simulink model "template_Final_Project_MPC5643L"  (Simulink 7.8)
settings: Solver=FixedStepDiscrete  StartTime=0.0  StopTime=10.0  RelTol=1e-3
InitFcn:
  | parameters
values from neighbouring files (symbols this model uses):
  Ak = 100    [parameters.m]
  b = 100    [parameters.m]
  dT = 0.01    [parameters.m]
  H = 10    [ACCLogic_TestCase1.m]    (also in ACCLogic_TestCase2.m)
  Kd_PD = 0.03    [parameters.m]
  Kd_PID = 75    [parameters.m]
  Ki_PID = 0.002    [parameters.m]
  Kp_PD = 0.4    [parameters.m]
  Kp_PID = 550    [parameters.m]
  m = 2000    [parameters.m]
  V_Ki = 50    [parameters.m]
  V_Kp = 5000    [parameters.m]
undefined symbols (not defined in the file or in its folder): A10, A13, A14, AN1, AN12, B, B13, B4, B6, C6, D, D11, D4, DiscIntNeverNeededParam, F15, F3, F4, G4, H4, L3, M14, N15, P7, PA10, PA11, PA12, PA13, PA14, PA5, PA6, PA7, PA8, PA9, PB10, PB8, PC11, PC12, PC13, PC14, PC6, PD11, R10, R16, R8
libraries: Conv_Lib x50, rappid_564xl_ec_toolbox x36, Veh_Sim x9, simulink x3, U_of_M_5643_blockset x1
(part 1 of 2)
settings Model: Creator=lab  LastModifiedBy=cjzhang
settings DataIOCC: ExternalInput=off  InitialState=off  SaveOutput=off  SignalLogging=off  SaveTime=off
settings OptimizationCC: InlineParams=on  OptimizeModelRefInitCode=on  LifeSpan=1
settings DebuggingCC: InheritedTsInSrcMsg=none  SingleTaskRateTransMsg=error  UnconnectedInputMsg=error  UnconnectedOutputMsg=error  UnconnectedLineMsg=error  FrameProcessingCompatibilityMsg=error  UnknownTsInhSupMsg=error
settings HardwareCC: ProdLargestAtomicInteger=Long  ProdLargestAtomicFloat=Double  ProdIntDivRoundTo=Zero  ProdEndianess=BigEndian  ProdHWDeviceType=Motorola PowerPC
settings RTWCC: SystemTargetFile=rappid564xl.tlc  MakeCommand=rappid_564xl_make_rtw  TemplateMakefile=rappid_564xl_default_tmf  PostCodeGenCommand=rappid_analyzegencode(buildInfo)  Description=RAppID Toolbox MPC564xL Code Generation Target (rappid)  GenerateReport=on  ProcessScript=rappid564xl_make_rtw_hook  IncludeHyperlinkInReport=on  LaunchReport=on
settings CodeAppCC: IgnoreCustomStorageClasses=off
settings STFCustomTargetCC: TargetFunctionLibrary=C89/C90 (ANSI)  GeneratePreprocessorConditionals=Use local settings  CombineOutputUpdateFcns=on  SuppressErrorStatus=on  ERTCustomFileBanners=on  SupportContinuousTime=off  SupportNonInlinedSFcns=off  SystemTargetFile=rappid564xl.tlc
settings ERTTargetCC: TargetFunctionLibrary=C89/C90 (ANSI)  MultiwordLength=2048  ParMdlRefBuildCompliant=off  CompOptLevelCompliant=off  ConcurrentExecutionCompliant=off  SuppressErrorStatus=on  ERTFirstTimeCompliant=off  ModelStepFunctionPrototypeControlCompliant=off  CPPClassGenCompliant=off  ExtModeMexFile=noextcomm  InlinedParameterPlacement=NonHierarchical  ERTCustomFileTemplate=example_file_process.tlc  ConvertIfToSwitch=off  SuppressUnreachableDefaultCases=off

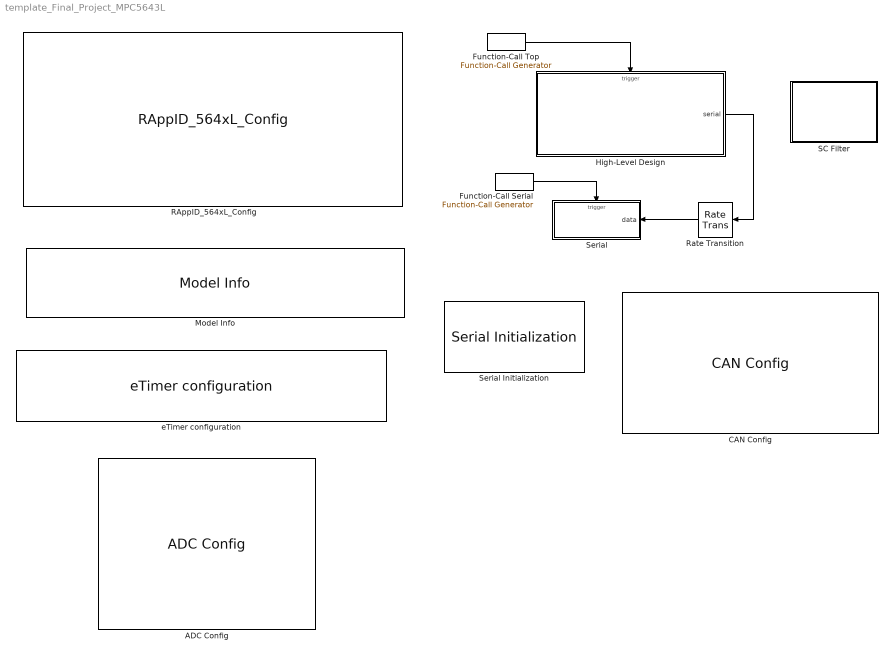
== system template_Final_Project_MPC5643L ==
  ADC Config : rappid_564xl_ec_toolbox/MPC564xL/Motor Control Blocks/ADC Config  adc_unit=0  adc_ctu=off  adc_owr=on  adc_wls=Left  adc_clk=on  adc_ack=on  adc_ctr0_inp=off  adc_ctr0_shft=10 - Avin = 0  adc_ctr0_cmp=01  adc_ctr0_samp=3  adc_ctr1_inp=off  adc_ctr1_cmp=01  adc_ctr1_samp=1  adc_ctr1_tsens=PTAT  adc_pscr_preval=V0  adc_pscr_preconv=off
  CAN Config : rappid_564xl_ec_toolbox/MPC564xL/Communication Blocks/CAN Config  Priority=1  can_unit=A  can_unit_v2=0  can_idam=A - One full ID (standard or extended) per filter element.  can_srx_dis=1 - Self reception disabled  can_presdiv=4  can_rjw=3  can_pseg1=5  can_pseg2=5  can_clk_src=0 - The CAN engine clock source is the oscillator clock  can_lpb=0 - Loop Back disabled  can_smp=0 - One sample is used to determine the bit value  can_boff_rec=0 - Automatic recovering from Bus Off state enabled  can_tsyn=0 - Timer Sync feature disabled  can_lbuf=0 - Buffer with highest priority is transmitted first  can_lom=0 - Listen Only Mode is deactivated  can_propseg=2
  Function-Call Serial : simulink/Ports & Subsystems/Function-Call Generator  sample_time=.05  numberOfIterations=1
  Function-Call Top : simulink/Ports & Subsystems/Function-Call Generator  sample_time=dT  numberOfIterations=1
  High-Level Design : Subsystem
  Model Info : simulink/Model-Wide Utilities/Model Info  InitialBlockCM=none  BlockCM=None  Frame=on  DisplayStringWithTags=|  HorizontalTextAlignment=Center  LeftAlignmentValue=0.5  SourceBlockDiagram=template_Final_Project_MPC5643L  TagMaxNumber=20
      | Model Notes:
      | 
      | You MUST change the CAN IDs whenever you change stations
      | 
      | First 2 buffers must be transmits
  RAppID_564xL_Config : rappid_564xl_ec_toolbox/MPC564xL/RAppID_564xL_Config  SystemClock=120  XTAL=40  MC_clock_60=12  MC_clock_80=16  MC_clock_120=10  SWG_clock_60=20  SWG_clock_80=13.334  SWG_clock_120=20  Compiler=CodeWarrior  MemTarget=FLASH  Part=MPC5643L  Package=144 LQFP  global_int_priority=10  base_tick_priority=11  sys_task_supress=off  exception_handlers=off  stored_mdl_name=adc_pit_block_new  freemaster_interface=Oops  freemaster_rx_pin="LINFlex_0 Rx Pin 116 : \"PB[3]\""  freemaster_tx_pin="LINFlex_0 Tx Pin 114 : \"PB[2]\""  freemaster_interface_1=Serial 0  freemaster_enable=on  freemaster_rate=115200  freemaster_tx0_pin=18 : B[2] : 114 : A14  freemaster_rx0_pin=19 : B[3] : 116 : B13  freemaster_tx1_pin=57 : D[9] : 26 : L3  freemaster_rx1_pin=29 : B[13] : 60 : R10  freemaster_can_channel=1CH  freemater_can_speed=500K  freemaster_can_msgig=0x7AA  ccp_interface=None  ccp_enable=off  ccp_can_channel=CH1 (MB 0 - 1)  ccp_can_speed=500K  ccp_can_cro_id=256  ccp_can_dto_id=257  ccp_dev_id=RappID  ccp_dev_addr=0  ccp_odt=3  ccp_daq=3  pil_enable=off  pil_bam=off  comport=4  pil_rate=115200  bam_password_def=on  bam_password=0xFEEDFACECAFEBEEF  bam_sa_cs=off  bam_start_address=0x0  bam_code_size=0x7000  cons_dspi=on  cons_can=on  cons_adc=on  cons_pwm=on  cons_ctu=on  cons_swg=on  cons_eTimer=on  cons_fm=on
  Rate Transition : RateTransition
  SC Filter : Subsystem
  Serial : Subsystem
  Serial Initialization : U_of_M_5643_blockset/Serial/Serial Initialization
  eTimer configuration : rappid_564xl_ec_toolbox/MPC564xL/Motor Control Blocks/eTimer configuration  SubModule=0  TimerChan=0  subMod=0  channel=0  CountMode=100 - Quadrature count mode using primary and secondary sources  CNTMODE=4  CountOnce=0 - Count repeatedly  ONCE=0  CountLength=0 - Continue counting to roll over  LENGTH=0  CountDirection=0 - Count up  DIR=0  OutputEnable=0 - The external pin is configured as an input  OEN=0  CoChanInit=00 - Other channels cannot force re-initialization of this channel  COINIT=0  StopAction=0 - Output enable is unaffected by stop mode  STPEN=0  ReloadOnCapt=00 - Do not reload the counter on a capture event  ROC=0  PrimarySource=00000 - Counter #0 input pin  PRISRC=0  PrimSrcPol=0 - True polarity  PIPS=0  SecondarySource=00001 - Counter #1 input pin  SECSRC=1  SecSrcPol=0 - True polarity  SIPS=0  FILT_CNT=0  FILT_PER=0  FILT=0  OutputMode=0000 - Software controlled  OUTMODE=0  OutputPol=0 - True polarity  OPS=0  MasterMode=0 - Disable broadcast of this channel output  MSTR=0  ForcedOutVal=0  VAL=0  CoForce=0 - Other channels cannot force this channel output  COFRC=0  CompLoad1=000 - COMP1 is never preload  CLC1=0  CompLoad2=000 - COMP2 is never preload  CLC2=0  CompareMode="00 - COMP1 and COMP2  are used when the counter is counting up"  CMPMODE=0  CaptMode1=00 - Capture disabled  CPT1MODE=0  CaptMode2=00 - Capture disabled  CPT2MODE=0  OneShCaptMode=0 - Free running mode is selected  ONESHOT=0  CaptFIFO=0  CFWM=0  CNTRinit=0  COMP1init=0  COMP2init=0  mod0ch0pin="0   : PA0  : [ 73 ] : [ T14 ]  input/output"  mod0ch1pin="1   : PA1  : [ 74 ] : [ R14 ]  input/output"  mod0ch2pin=None  mod0ch3pin=None  mod0ch4pin=None  mod0ch5pin=None  mod1ch0pin=None  mod1ch1pin=None  mod1ch2pin=None  mod1ch3pin=None  mod1ch4pin=None  mod1ch5pin=None  mod2ch0pin=None  mod2ch1pin=None  mod2ch2pin=None  mod2ch3pin=None  mod2ch4pin=None  mod2ch5pin=None  pcrNum0=0  pcrNum1=1  pcrNum2=255  pcrNum3=255  pcrNum4=255  pcrNum5=255  TCFIE=off  TCF1IE=off  TCF2IE=off  TOFIE=off  IELFIE=off  IEHFIE=off  ICF1IE=off  ICF2IE=off  INTDMA=0
  wires:
  Function-Call Serial/1 -> Serial/Trigger
  Rate Transition/1 -> Serial/1(data)
  Function-Call Top/1 -> High-Level Design/Trigger
  High-Level Design/1(serial) -> Rate Transition/1

== system template_Final_Project_MPC5643L/High-Level Design ==
  Trigger : TriggerPort  TriggerType=function-call
  Automatic Cruise Control : Subsystem
  Automatic Steering : Subsystem
  Inputs : Subsystem
  Outputs : Subsystem
  Unit Delay : UnitDelay  SampleTime=-1
  Vehicle Model : Subsystem
  serial : Outport
  wires:
  Outputs/1(x,y,psi (Cars 1 - 6)) -> serial/1
  Vehicle Model/3(u  (This Car)) -> Outputs/3(u (This Car))
  Inputs/1(s,n,psi,us (Cars 1 - 6)) -> Outputs/1(s,n,psi,us (Cars 1 - 6)), Automatic Cruise Control/1(s,n,psi,us (Cars 1 - 6))
  Vehicle Model/2(s,n,psi,us (This Car)) -> Outputs/2(s,n,psi,us (This Car)), Unit Delay/1
  Automatic Steering/1(Auto Torque) -> Outputs/5(Auto torque)
  Inputs/3(Cruise Control Speed) -> Automatic Cruise Control/3(Cruise Control Speed)
  Inputs/2(ACC_enable) -> Automatic Cruise Control/2("ACC_enable ")
  Inputs/4(Steering Angle (delta)) -> Automatic Cruise Control/4(Steering Angle (delta)), Automatic Steering/3(delta)
  Inputs/5(Throttle (Fd)) -> Automatic Cruise Control/5(Throttle (Fd))
  Inputs/6(Automatic Steering_enable) -> Automatic Steering/1(Automatic Steering_enable)
  Vehicle Model/1(Self-aligning torque) -> Outputs/4(Self-aligning torque)
  Unit Delay/1 -> Automatic Cruise Control/6(s,n,psi,us (This Car)), Automatic Steering/2(s,n,psi,us (This Car))
  Automatic Cruise Control/1(Force) -> Vehicle Model/1("Force ")
  Automatic Cruise Control/2(delta) -> Vehicle Model/2(delta)

== system template_Final_Project_MPC5643L/SC Filter ==
  Constant1 : Constant  Value=1e6  OutDataTypeStr=uint32
  Constant2 : Constant  Value=0  OutDataTypeStr=uint32
  Constant3 : Constant  Value=50  OutDataTypeStr=uint32
  Simple PWM Output : rappid_564xl_ec_toolbox/MPC564xL/Motor Control Blocks/Simple PWM Output  Priority=1  pwmModule=0  pwmMod=0  SubModule=1  subMod=1  InitFreq=1000000  resolution=1 %  resValue=1  InitDutyA=0  InitDutyB=50  align=A B - edge aligned  PhaseShift_A=0  PhaseShift=0  Phase_A=0  Phase_B=0  centered=0  DoubleS=off  doubleSw=off  debugSw=off  debug_mode=0  pin_A0=None  pin_B0=None  pin_X0=None  pin_A1=None  pin_B1="38  : PC6  : [ 142 ] : [ D4 ]"  pin_X1=None  pin_A2=None  pin_B2=None  pin_X2=None  pin_A3=None  pin_B3=None  pin_X3=None  pin1_A0=None  pin1_B0=None  pin1_X0=None  pin1_A1=None  pin1_B1=None  pin1_X1=None  pin1_A2=None  pin1_B2=None  pin1_X2=None  pin1_A3=None  pin1_B3=None  pin1_X3=None  pcrNumA=255  pcrNumB=38  pcrNumX=255  polA=off  polB=off  polX=off  octrl=0  syncFrom0=off  masterSync=0  outVal0=off  outVal1=off  outVal2=off  outVal3=off  outVal4=on  outVal5=on  outTrig=48
  wires:
  Constant1/1 -> Simple PWM Output/1
  Constant2/1 -> Simple PWM Output/2
  Constant3/1 -> Simple PWM Output/3

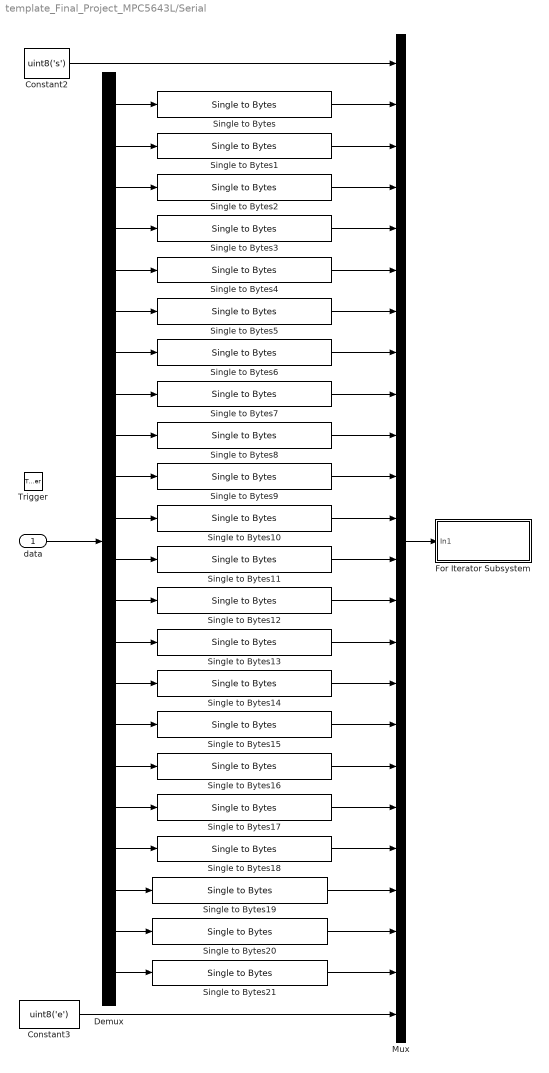
== system template_Final_Project_MPC5643L/Serial ==
  data : Inport
  Trigger : TriggerPort  TriggerType=function-call
  Constant2 : Constant  Value=uint8('s')  OutDataTypeStr=uint8
  Constant3 : Constant  Value=uint8('e')  OutDataTypeStr=uint8
  Demux : Demux  Outputs=22
  For Iterator Subsystem : Subsystem
  Mux : Mux  Inputs=24
  Single to Bytes{,1..21} (22 alike) : Conv_Lib/Single to Bytes
  wires:
  Constant2/1 -> Mux/1
  Single to Bytes/1 -> Mux/2
  Single to Bytes1/1 -> Mux/3
  Single to Bytes2/1 -> Mux/4
  Single to Bytes3/1 -> Mux/5
  Single to Bytes4/1 -> Mux/6
  Single to Bytes5/1 -> Mux/7
  Single to Bytes6/1 -> Mux/8
  Single to Bytes7/1 -> Mux/9
  Single to Bytes8/1 -> Mux/10
  Single to Bytes9/1 -> Mux/11
  Single to Bytes10/1 -> Mux/12
  Single to Bytes11/1 -> Mux/13
  Single to Bytes12/1 -> Mux/14
  Single to Bytes13/1 -> Mux/15
  Single to Bytes15/1 -> Mux/17
  Single to Bytes16/1 -> Mux/18
  Single to Bytes17/1 -> Mux/19
  Mux/1 -> For Iterator Subsystem/1(In1)
  Demux/1 -> Single to Bytes/1
  Demux/2 -> Single to Bytes1/1
  Demux/3 -> Single to Bytes2/1
  Demux/4 -> Single to Bytes3/1
  Demux/5 -> Single to Bytes4/1
  Demux/6 -> Single to Bytes5/1
  Demux/7 -> Single to Bytes6/1
  Demux/8 -> Single to Bytes7/1
  Demux/9 -> Single to Bytes8/1
  Demux/10 -> Single to Bytes9/1
  Demux/11 -> Single to Bytes10/1
  Demux/12 -> Single to Bytes11/1
  Demux/13 -> Single to Bytes12/1
  Demux/14 -> Single to Bytes13/1
  Demux/15 -> Single to Bytes14/1
  Demux/16 -> Single to Bytes15/1
  Demux/17 -> Single to Bytes16/1
  Demux/18 -> Single to Bytes17/1
  data/1 -> Demux/1
  Single to Bytes14/1 -> Mux/16
  Demux/19 -> Single to Bytes18/1
  Demux/20 -> Single to Bytes19/1
  Demux/21 -> Single to Bytes20/1
  Demux/22 -> Single to Bytes21/1
  Single to Bytes18/1 -> Mux/20
  Single to Bytes19/1 -> Mux/21
  Single to Bytes20/1 -> Mux/22
  Single to Bytes21/1 -> Mux/23
  Constant3/1 -> Mux/24

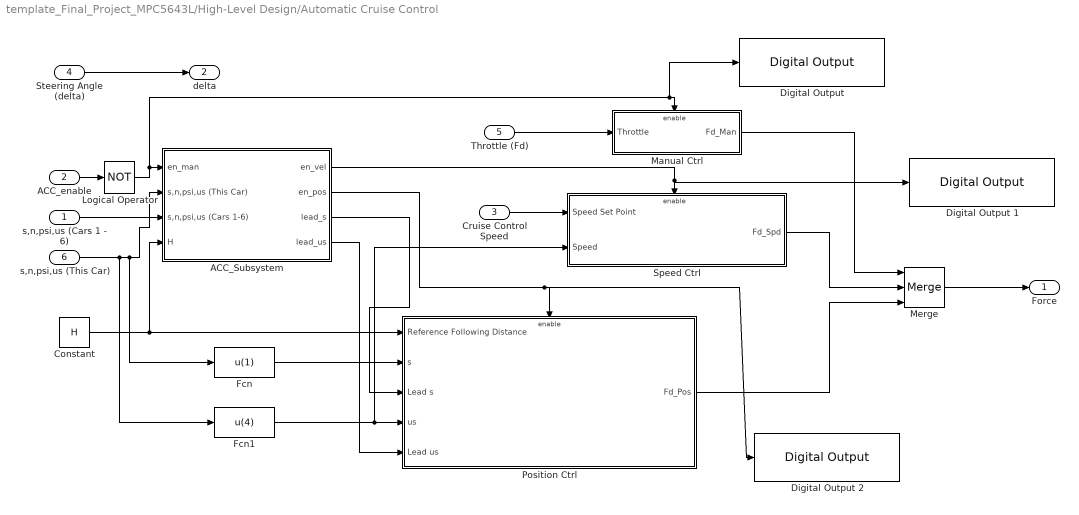
== system template_Final_Project_MPC5643L/High-Level Design/Automatic Cruise Control ==
  s,n,psi,us (Cars 1 - 6) : Inport
  "ACC_enable " : Inport  Port=2
  Cruise Control Speed : Inport  Port=3
  Steering Angle (delta) : Inport  Port=4
  Throttle (Fd) : Inport  Port=5
  s,n,psi,us (This Car) : Inport  Port=6
  ACC_Subsystem : Subsystem
  Constant : Constant  Value=H  OutDataTypeStr=single
  "Digital Output " : rappid_564xl_ec_toolbox/MPC564xL/General Purpose Blocks/Digital Output   gpio_outputs="43  : PC11 : [ 80 ] : [ M14 ]"  pinNum=[ 80 ]  pcrNum=43
  Digital Output 1 : rappid_564xl_ec_toolbox/MPC564xL/General Purpose Blocks/Digital Output   gpio_outputs="44  : PC12 : [ 82 ] : [ N15 ]"  pinNum=[ 82 ]  pcrNum=44
  Digital Output 2 : rappid_564xl_ec_toolbox/MPC564xL/General Purpose Blocks/Digital Output   gpio_outputs="45  : PC13 : [ 101 ] : [ F15 ]"  pinNum=[ 101 ]  pcrNum=45
  Fcn : Fcn  Expr=u(1)
  Fcn1 : Fcn  Expr=u(4)
  Logical Operator : Logic  Operator=NOT  AllPortsSameDT=off  OutDataTypeStr=boolean
  Manual Ctrl : Subsystem  TreatAsAtomicUnit=on
  Merge : Merge  Inputs=3
  Position Ctrl : Subsystem  TreatAsAtomicUnit=on
  Speed Ctrl : Subsystem  TreatAsAtomicUnit=on
  Force : Outport
  delta : Outport  Port=2
  wires:
  Steering Angle (delta)/1 -> delta/1
  Cruise Control Speed/1 -> Speed Ctrl/1(Speed Set Point)
  Speed Ctrl/1(Fd_Spd) -> Merge/2
  Position Ctrl/1(Fd_Pos) -> Merge/3
  Fcn/1 -> Position Ctrl/2(s)
  Fcn1/1 -> Position Ctrl/4(us), Speed Ctrl/2(Speed)
  Constant/1 -> Position Ctrl/1(Reference Following Distance), ACC_Subsystem/4(H)
  Throttle (Fd)/1 -> Manual Ctrl/1(Throttle)
  Manual Ctrl/1(Fd_Man) -> Merge/1
  Merge/1 -> Force/1
  "ACC_enable "/1 -> Logical Operator/1
  s,n,psi,us (This Car)/1 -> ACC_Subsystem/2(s,n,psi,us (This Car)), Fcn/1, Fcn1/1
  s,n,psi,us (Cars 1 - 6)/1 -> ACC_Subsystem/3(s,n,psi,us (Cars 1-6))
  Logical Operator/1 -> ACC_Subsystem/1(en_man), Manual Ctrl/Enable, "Digital Output "/1
  ACC_Subsystem/2(en_pos) -> Position Ctrl/Enable, Digital Output 2/1
  ACC_Subsystem/3(lead_s) -> Position Ctrl/3(Lead s)
  ACC_Subsystem/4(lead_us) -> Position Ctrl/5(Lead us)
  ACC_Subsystem/1(en_vel) -> Speed Ctrl/Enable, Digital Output 1/1

== system template_Final_Project_MPC5643L/High-Level Design/Automatic Steering ==
  Automatic Steering_enable : Inport
  s,n,psi,us (This Car) : Inport  Port=2
  delta : Inport  Port=3
  Automatic Steering : Subsystem  TreatAsAtomicUnit=on
  Constant1 : Constant  Value=0  OutDataTypeStr=single
  Digital Output 3 : rappid_564xl_ec_toolbox/MPC564xL/General Purpose Blocks/Digital Output   gpio_outputs="46  : PC14 : [ 103 ] : [ E15 ]"  pinNum=[ 103 ]  pcrNum=46
  Switch : Switch  Criteria=u2 > Threshold
  Auto Torque : Outport
  wires:
  Automatic Steering_enable/1 -> Automatic Steering/Enable, Switch/2, Digital Output 3/1
  s,n,psi,us (This Car)/1 -> Automatic Steering/1(s,n,psi,us (This Car))
  delta/1 -> Automatic Steering/2(delta)
  Constant1/1 -> Switch/3
  Automatic Steering/1(auto_torque) -> Switch/1
  Switch/1 -> Auto Torque/1

== system template_Final_Project_MPC5643L/High-Level Design/Inputs ==
  ADC Channel1 : rappid_564xl_ec_toolbox/MPC564xL/Motor Control Blocks/ADC Channel  adc_unit=0  adc_chan0=older  adc_chan0_v2=24 : PB8 : [47] : [P7] : AN1  adc_chan1=older  adc_chan1_v2=26 : PB10 : [53] : [R8] : AN12  simulate=off  interrupt=off  adc_mode=Normal  adc_presample=off
  Constant1 : Constant  Value=50  OutDataTypeStr=single
  Digital Input : rappid_564xl_ec_toolbox/MPC564xL/General Purpose Blocks/Digital Input  gpio_outputs="13  : PA13 : [ 136 ] : [ C6 ]"  pinNum=[ 136 ]  pcrNum=13
  Digital Input1 : rappid_564xl_ec_toolbox/MPC564xL/General Purpose Blocks/Digital Input  gpio_outputs="14  : PA14 : [ 143 ] : [ B4 ]"  pinNum=[ 143 ]  pcrNum=14
  Haptic Wheel Input : Subsystem
  Other Cars : Subsystem
  Read 8 bits : Subsystem
  Sum : Sum  Inputs=+|-
  s,n,psi,us (Cars 1 - 6) : Outport
  ACC_enable : Outport  Port=2
  Cruise Control Speed : Outport  Port=3
  Steering Angle (delta) : Outport  Port=4
  Throttle (Fd) : Outport  Port=5
  Automatic Steering_enable : Outport  Port=6
  wires:
  Digital Input1/1 -> Automatic Steering_enable/1
  Other Cars/1(s,n,psi,us (Car 1 - 6)) -> s,n,psi,us (Cars 1 - 6)/1
  Digital Input/1 -> ACC_enable/1
  Haptic Wheel Input/1(Haptic Wheel Position (radians)) -> Steering Angle (delta)/1
  Read 8 bits/1(8 bits) -> Cruise Control Speed/1
  ADC Channel1/1 -> Sum/1
  Sum/1 -> Throttle (Fd)/1
  Constant1/1 -> Sum/2

== system template_Final_Project_MPC5643L/High-Level Design/Outputs ==
  s,n,psi,us (Cars 1 - 6) : Inport
  s,n,psi,us (This Car) : Inport  Port=2
  u (This Car) : Inport  Port=3
  Self-aligning torque : Inport  Port=4
  Auto torque : Inport  Port=5
  Extract x,y,psi : Subsystem
  Extract x,y,psi (Cars 1 - 6) : Subsystem
  Mux : Mux  Inputs=3
  Subsystem : Subsystem
  Sum : Sum  Inputs=+|+
  Tx CAN : Subsystem
  x,y,psi (Cars 1 - 6) : Outport
  wires:
  s,n,psi,us (Cars 1 - 6)/1 -> Extract x,y,psi (Cars 1 - 6)/1(s,n,psi,us (Cars 1 - 6))
  s,n,psi,us (This Car)/1 -> Extract x,y,psi/1(s,n,psi,us), Tx CAN/1(s,n,psi,us)
  Extract x,y,psi/1(x,y,psi) -> Mux/1
  Mux/1 -> x,y,psi (Cars 1 - 6)/1
  u (This Car)/1 -> Mux/2
  Extract x,y,psi (Cars 1 - 6)/1(x,y,psi (Cars 1 - 6)) -> Mux/3
  Self-aligning torque/1 -> Sum/1
  Auto torque/1 -> Sum/2
  Sum/1 -> Subsystem/1(Torque)

== system template_Final_Project_MPC5643L/High-Level Design/Vehicle Model ==
  "Force " : Inport
  delta : Inport  Port=2
  Gain : Gain  Gain=Ak
  Look up Forward Vector : Veh_Sim/Look up Forward Vector  SystemSampleTime=-1
  Mux : Mux
  Product : Product  RndMeth=Zero
  S-Function Builder : S-Function  InitFcn=try, set_param(gcb,'FunctionName','us_calc'), end  FunctionName=us_calc  SFunctionModules=us_calc_wrapper  WizardData=DataTag0  EnableBusSupport=off  mask(S-Function Builder){}
      mask help: Simulink:masks:SFunctionBuilder_MD
      mask init:
      | val = [[.9  0.75 0.75 1 1 .9 .9 1]',[1 1 0.75 0.75 .9 .9 1 .9]'];try , sys = get_param(gcb,'SfunBuilderFcnName');if isempty(sys), sys = get_param(gcb,'FunctionName'); end,catch, sys = get_param(gcb,'FunctionName'); end
      settings: CopyFcn=set_param(gcbh,'LinkStatus','none')  PreSaveFcn=try, set_param(gcb,'FunctionName','us_calc'), end  OpenFcn=sfunctionwizard(gcbh)
      mask Display: plot(val(:,1),val(:,2)),disp(sys), port_label('input',1,'delta'), port_label('input',2,'psi'), port_label('input',3,'fx'), port_label('input',4,'fy'), port_label('input',5,'u'), port_label('output',1,'us')
  Vehicle Dynamics : Subsystem  TreatAsAtomicUnit=on
  x,y to s,n : Veh_Sim/x,y to s,n  SystemSampleTime=-1
  Self-aligning torque : Outport
  s,n,psi,us (This Car) : Outport  Port=2
  u  (This Car) : Outport  Port=3
  wires:
  "Force "/1 -> Vehicle Dynamics/1(Fd)
  delta/1 -> Vehicle Dynamics/2(delta), Product/2, S-Function Builder/1
  Vehicle Dynamics/3(u) -> Product/1, u  (This Car)/1, S-Function Builder/5
  Gain/1 -> Self-aligning torque/1
  Product/1 -> Gain/1
  Vehicle Dynamics/1(x) -> x,y to s,n/1
  Vehicle Dynamics/2(y) -> x,y to s,n/2
  x,y to s,n/1 -> Mux/1, Look up Forward Vector/1
  x,y to s,n/2 -> Mux/2
  Vehicle Dynamics/4(psi) -> Mux/3, S-Function Builder/2
  Look up Forward Vector/1 -> S-Function Builder/3
  Look up Forward Vector/2 -> S-Function Builder/4
  S-Function Builder/1 -> Mux/4
  Mux/1 -> s,n,psi,us (This Car)/1

== system template_Final_Project_MPC5643L/Serial/For Iterator Subsystem ==
  In1 : Inport
  Data Type Conversion : DataTypeConversion  OutDataTypeStr=uint8
  For Iterator : ForIterator  IterationLimit=91  IndexMode=Zero-based  IterationVariableDataType=int8
  Index Vector : MultiPortSwitch  DataPortOrder=Zero-based contiguous  Inputs=1  zeroidx=on
  S-Function : S-Function  FunctionName=SerialSend  EnableBusSupport=off
  wires:
  In1/1 -> Index Vector/2
  Index Vector/1 -> Data Type Conversion/1
  For Iterator/1 -> Index Vector/1
  Data Type Conversion/1 -> S-Function/1

== system template_Final_Project_MPC5643L/High-Level Design/Automatic Cruise Control/ACC_Subsystem ==
  en_man : Inport
  s,n,psi,us (This Car) : Inport  Port=2
  s,n,psi,us (Cars 1-6) : Inport  Port=3
  H : Inport  Port=4
  S-Function Builder : S-Function  InitFcn=try, set_param(gcb,'FunctionName','ACC_Logic'), end  FunctionName=ACC_Logic  SFunctionModules=ACC_Logic_wrapper  EnableBusSupport=off
      mask init: same as template_Final_Project_MPC5643L/High-Level Design/Vehicle Model/S-Function Builder
      settings: CopyFcn=set_param(gcbh,'LinkStatus','none')  PreSaveFcn=try, set_param(gcb,'FunctionName','ACC_Logic'), end  OpenFcn=sfunctionwizard(gcbh)
      mask Display: plot(val(:,1),val(:,2)),disp(sys), port_label('input',1,'en_man'), port_label('input',2,'s'), port_label('input',3,'u'), port_label('input',4,'H'), port_label('output',1,'en_vel'), port_label('output',2,'en_pos'), port_label('output',3,'lead_s'), port_label('output',4,'lead_us')
  Subsystem : Subsystem
  Subsystem1 : Subsystem
  en_vel : Outport
  en_pos : Outport  Port=2
  lead_s : Outport  Port=3
  lead_us : Outport  Port=4
  wires:
  en_man/1 -> S-Function Builder/1
  s,n,psi,us (This Car)/1 -> Subsystem/1(s,n,psi,us (This Car)), Subsystem1/1(s,n,psi,us (This Car))
  s,n,psi,us (Cars 1-6)/1 -> Subsystem/2(s,n,psi,us (Cars 1-6)), Subsystem1/2(s,n,psi,us (Cars 1-6))
  Subsystem/1(s) -> S-Function Builder/2
  S-Function Builder/2 -> en_pos/1
  S-Function Builder/3 -> lead_s/1
  Subsystem1/1(u) -> S-Function Builder/3
  H/1 -> S-Function Builder/4
  S-Function Builder/4 -> lead_us/1
  S-Function Builder/1 -> en_vel/1

== system template_Final_Project_MPC5643L/High-Level Design/Automatic Cruise Control/Manual Ctrl ==
  Throttle : Inport
  Enable : EnablePort
  Fd_Man : Outport
  wires:
  Throttle/1 -> Fd_Man/1  "desired speed"

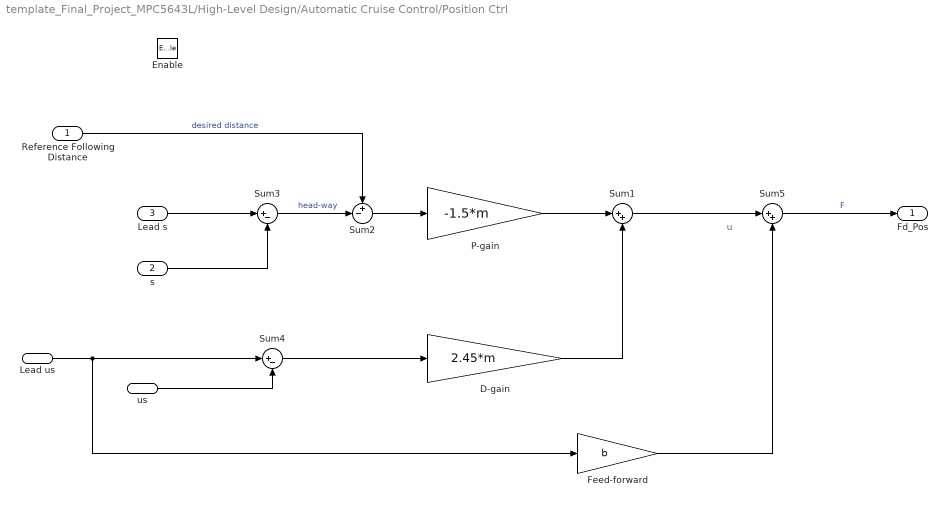
== system template_Final_Project_MPC5643L/High-Level Design/Automatic Cruise Control/Position Ctrl ==
  note: u
  Reference Following Distance : Inport
  s : Inport  Port=2
  Lead s : Inport  Port=3
  us : Inport  Port=4
  Lead us : Inport  Port=5
  Enable : EnablePort
  D-gain : Gain  Gain=2.45*m  SaturateOnIntegerOverflow=on  OutDataTypeStr=Inherit: Same as input  ParamDataTypeStr=Inherit: Same as input
  Feed-forward : Gain  Gain=b  SaturateOnIntegerOverflow=on  OutDataTypeStr=Inherit: Same as input  ParamDataTypeStr=Inherit: Same as input
  P-gain : Gain  Gain=-1.5*m  SaturateOnIntegerOverflow=on  OutDataTypeStr=Inherit: Same as input  ParamDataTypeStr=Inherit: Same as input
  Sum1 : Sum  Inputs=|++  SaturateOnIntegerOverflow=on
  Sum2 : Sum  Inputs=+-|  SaturateOnIntegerOverflow=on
  Sum3 : Sum  Inputs=|+-  SaturateOnIntegerOverflow=on
  Sum4 : Sum  Inputs=|+-  SaturateOnIntegerOverflow=on
  Sum5 : Sum  Inputs=|++  SaturateOnIntegerOverflow=on
  Fd_Pos : Outport
  wires:
  Sum1/1 -> Sum5/1
  Sum5/1 -> Fd_Pos/1  "F"
  Feed-forward/1 -> Sum5/2
  Sum4/1 -> D-gain/1
  Lead us/1 -> Feed-forward/1, Sum4/1
  us/1 -> Sum4/2
  D-gain/1 -> Sum1/2
  P-gain/1 -> Sum1/1
  Sum2/1 -> P-gain/1
  Sum3/1 -> Sum2/2  "head-way"
  Reference Following Distance/1 -> Sum2/1  "desired distance"
  s/1 -> Sum3/2
  Lead s/1 -> Sum3/1

== system template_Final_Project_MPC5643L/High-Level Design/Automatic Cruise Control/Speed Ctrl ==
  Speed Set Point : Inport
  Speed : Inport  Port=2
  Enable : EnablePort
  Gain : Gain  Gain=b  SaturateOnIntegerOverflow=on  OutDataTypeStr=Inherit: Same as input  ParamDataTypeStr=Inherit: Same as input
  PI : Subsystem
  Sum : Sum  Inputs=++|  SaturateOnIntegerOverflow=on
  Sum1 : Sum  Inputs=|+-  SaturateOnIntegerOverflow=on
  Fd_Spd : Outport
  wires:
  PI/1(U) -> Sum/2
  Gain/1 -> Sum/1
  Sum1/1 -> PI/1(Error)
  Speed/1 -> Sum1/2
  Speed Set Point/1 -> Sum1/1, Gain/1  "desired speed"
  Sum/1 -> Fd_Spd/1  "Fd"

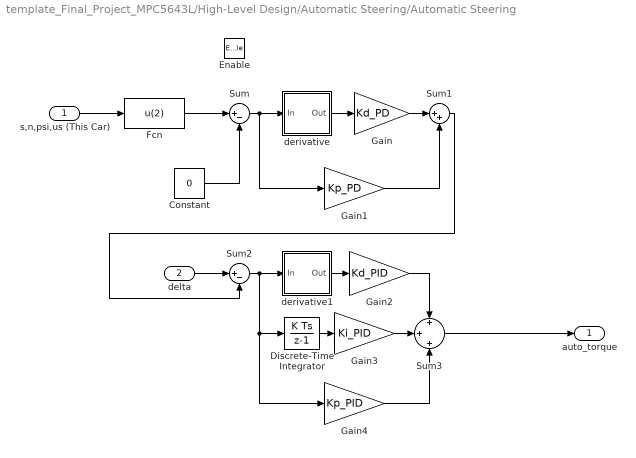
== system template_Final_Project_MPC5643L/High-Level Design/Automatic Steering/Automatic Steering ==
  s,n,psi,us (This Car) : Inport
  delta : Inport  Port=2
  Enable : EnablePort
  Constant : Constant  Value=0  OutDataTypeStr=single
  Discrete-Time Integrator : DiscreteIntegrator  SampleTime=-1  ICPrevOutput=DiscIntNeverNeededParam  ICPrevScaledInput=DiscIntNeverNeededParam
  Fcn : Fcn  Expr=u(2)
  Gain : Gain  Gain=Kd_PD
  Gain1 : Gain  Gain=Kp_PD
  Gain2 : Gain  Gain=Kd_PID
  Gain3 : Gain  Gain=Ki_PID
  Gain4 : Gain  Gain=Kp_PID
  Sum : Sum  Inputs=|+-
  Sum1 : Sum  Inputs=|++
  Sum2 : Sum  Inputs=|+-
  Sum3 : Sum  Inputs=+|+|+
  derivative : Subsystem
  derivative1 : Subsystem
  auto_torque : Outport
  wires:
  Sum/1 -> Gain1/1, derivative/1(In)
  Gain/1 -> Sum1/1
  Gain1/1 -> Sum1/2
  Sum2/1 -> Gain4/1, Discrete-Time Integrator/1, derivative1/1(In)
  Gain3/1 -> Sum3/2
  Gain2/1 -> Sum3/1
  Gain4/1 -> Sum3/3
  derivative1/1(Out) -> Gain2/1
  Discrete-Time Integrator/1 -> Gain3/1
  Constant/1 -> Sum/2
  derivative/1(Out) -> Gain/1
  Fcn/1 -> Sum/1
  s,n,psi,us (This Car)/1 -> Fcn/1
  Sum1/1 -> Sum2/2
  delta/1 -> Sum2/1
  Sum3/1 -> auto_torque/1

== system template_Final_Project_MPC5643L/High-Level Design/Inputs/Haptic Wheel Input ==
  Gain : Gain  Gain=-1
  Subsystem : Subsystem
  eTimer CNTR Register Read : rappid_564xl_ec_toolbox/MPC564xL/Motor Control Blocks/eTimer CNTR Register Read  SubModule=0  TimerChan=0  subMod=0  channel=0
  Haptic Wheel Position (radians) : Outport
  wires:
  eTimer CNTR Register Read/1 -> Subsystem/1(encoder counts)
  Subsystem/1(Haptic  Wheel  Position  (radians)) -> Gain/1
  Gain/1 -> Haptic Wheel Position (radians)/1

== system template_Final_Project_MPC5643L/High-Level Design/Inputs/Other Cars ==
  "0 for GSI vehicle only, 1 for ALL student vehicles" : Constant  OutDataTypeStr=single
  GSI Car : Subsystem
  GSI Car1 : Subsystem
  GSI Car2 : Subsystem
  GSI Car3 : Subsystem
  GSI Car4 : Subsystem
  GSI Car5 : Subsystem
  Mux1 : Mux  Inputs=6
  Switch : Switch  Criteria=u2 ~= 0
  s,n,psi,us (Car 1 - 6) : Outport
  wires:
  GSI Car/1(s,n,psi,us) -> Mux1/1
  Mux1/1 -> Switch/1, Switch/3
  Switch/1 -> s,n,psi,us (Car 1 - 6)/1
  "0 for GSI vehicle only, 1 for ALL student vehicles"/1 -> Switch/2
  GSI Car1/1(s,n,psi,us) -> Mux1/2
  GSI Car2/1(s,n,psi,us) -> Mux1/3
  GSI Car3/1(s,n,psi,us) -> Mux1/4
  GSI Car4/1(s,n,psi,us) -> Mux1/5
  GSI Car5/1(s,n,psi,us) -> Mux1/6

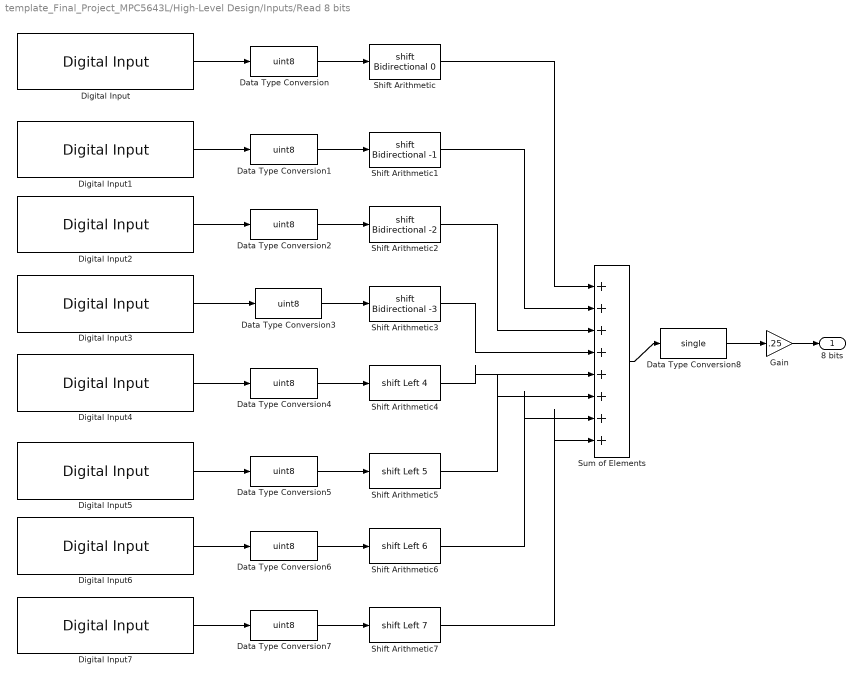
== system template_Final_Project_MPC5643L/High-Level Design/Inputs/Read 8 bits ==
  Data Type Conversion{,1..7} (8 alike) : DataTypeConversion  OutDataTypeStr=uint8
  Data Type Conversion8 : DataTypeConversion  OutDataTypeStr=single
  Digital Input : rappid_564xl_ec_toolbox/MPC564xL/General Purpose Blocks/Digital Input  gpio_outputs="5   : PA5  : [ 14 ] : [ H4 ]"  pinNum=[ 14 ]  pcrNum=5
  Digital Input1 : rappid_564xl_ec_toolbox/MPC564xL/General Purpose Blocks/Digital Input  gpio_outputs="6   : PA6  : [ 2 ] : [ G4 ]"  pinNum=[ 2 ]  pcrNum=6
  Digital Input2 : rappid_564xl_ec_toolbox/MPC564xL/General Purpose Blocks/Digital Input  gpio_outputs="7   : PA7  : [ 10 ] : [ F3 ]"  pinNum=[ 10 ]  pcrNum=7
  Digital Input3 : rappid_564xl_ec_toolbox/MPC564xL/General Purpose Blocks/Digital Input  gpio_outputs="8   : PA8  : [ 12 ] : [ F4 ]"  pinNum=[ 12 ]  pcrNum=8
  Digital Input4 : rappid_564xl_ec_toolbox/MPC564xL/General Purpose Blocks/Digital Input  gpio_outputs="9   : PA9  : [ 134 ] : [ B6 ]"  pinNum=[ 134 ]  pcrNum=9
  Digital Input5 : rappid_564xl_ec_toolbox/MPC564xL/General Purpose Blocks/Digital Input  gpio_outputs="10  : PA10  : [ 118 ] : [ A13 ]"  pinNum=[ 118 ]  pcrNum=10
  Digital Input6 : rappid_564xl_ec_toolbox/MPC564xL/General Purpose Blocks/Digital Input  gpio_outputs="11  : PA11 : [ 120 ] : [ D11 ]"  pinNum=[ 120 ]  pcrNum=11
  Digital Input7 : rappid_564xl_ec_toolbox/MPC564xL/General Purpose Blocks/Digital Input  gpio_outputs="12  : PA12 : [ 122 ] : [ A10 ]"  pinNum=[ 122 ]  pcrNum=12
  Gain : Gain  Gain=.25
  Shift Arithmetic : ArithShift
  Shift Arithmetic1 : ArithShift  BitShiftNumber=-1
  Shift Arithmetic2 : ArithShift  BitShiftNumber=-2
  Shift Arithmetic3 : ArithShift  BitShiftNumber=-3
  Shift Arithmetic4 : ArithShift  BitShiftNumber=4  BitShiftDirection=Left
  Shift Arithmetic5 : ArithShift  BitShiftNumber=5  BitShiftDirection=Left
  Shift Arithmetic6 : ArithShift  BitShiftNumber=6  BitShiftDirection=Left
  Shift Arithmetic7 : ArithShift  BitShiftNumber=7  BitShiftDirection=Left
  Sum of Elements : Sum  Inputs=|+|+|+|+|+|+|+|+  OutDataTypeStr=single
  8 bits : Outport
  wires:
  Digital Input/1 -> Data Type Conversion/1
  Digital Input1/1 -> Data Type Conversion1/1
  Digital Input2/1 -> Data Type Conversion2/1
  Digital Input3/1 -> Data Type Conversion3/1
  Data Type Conversion/1 -> Shift Arithmetic/1
  Data Type Conversion1/1 -> Shift Arithmetic1/1
  Data Type Conversion2/1 -> Shift Arithmetic2/1
  Data Type Conversion3/1 -> Shift Arithmetic3/1
  Shift Arithmetic1/1 -> Sum of Elements/2
  Shift Arithmetic2/1 -> Sum of Elements/3
  Shift Arithmetic3/1 -> Sum of Elements/4
  Digital Input4/1 -> Data Type Conversion4/1
  Digital Input5/1 -> Data Type Conversion5/1
  Digital Input6/1 -> Data Type Conversion6/1
  Digital Input7/1 -> Data Type Conversion7/1
  Data Type Conversion4/1 -> Shift Arithmetic4/1
  Data Type Conversion5/1 -> Shift Arithmetic5/1
  Data Type Conversion6/1 -> Shift Arithmetic6/1
  Data Type Conversion7/1 -> Shift Arithmetic7/1
  Shift Arithmetic4/1 -> Sum of Elements/5
  Shift Arithmetic5/1 -> Sum of Elements/6
  Shift Arithmetic6/1 -> Sum of Elements/7
  Shift Arithmetic7/1 -> Sum of Elements/8
  Shift Arithmetic/1 -> Sum of Elements/1
  Gain/1 -> 8 bits/1
  Sum of Elements/1 -> Data Type Conversion8/1
  Data Type Conversion8/1 -> Gain/1

== system template_Final_Project_MPC5643L/High-Level Design/Outputs/Extract x,y,psi ==
  s,n,psi,us : Inport
  Demux : Demux
  Mux : Mux  Inputs=3
  Terminator : Terminator
  s,n to x,y : Veh_Sim/s,n to x,y  SystemSampleTime=-1
  x,y,psi : Outport
  wires:
  Demux/1 -> s,n to x,y/1
  Demux/2 -> s,n to x,y/2
  s,n,psi,us/1 -> Demux/1
  s,n to x,y/1 -> Mux/1
  s,n to x,y/2 -> Mux/2
  Demux/3 -> Mux/3
  Demux/4 -> Terminator/1
  Mux/1 -> x,y,psi/1

== system template_Final_Project_MPC5643L/High-Level Design/Outputs/Extract x,y,psi (Cars 1 - 6) ==
  s,n,psi,us (Cars 1 - 6) : Inport
  Demux : Demux  Outputs=6
  Extract x,y,psi : Subsystem
  Extract x,y,psi1 : Subsystem
  Extract x,y,psi2 : Subsystem
  Extract x,y,psi3 : Subsystem
  Extract x,y,psi4 : Subsystem
  Extract x,y,psi5 : Subsystem
  Mux : Mux  Inputs=6
  x,y,psi (Cars 1 - 6) : Outport
  wires:
  Demux/1 -> Extract x,y,psi/1(s,n,psi,us)
  Extract x,y,psi/1(x,y,psi) -> Mux/1
  Demux/2 -> Extract x,y,psi1/1(s,n,psi,us)
  Extract x,y,psi1/1(x,y,psi) -> Mux/2
  Demux/3 -> Extract x,y,psi2/1(s,n,psi,us)
  Extract x,y,psi2/1(x,y,psi) -> Mux/3
  Demux/4 -> Extract x,y,psi3/1(s,n,psi,us)
  Extract x,y,psi3/1(x,y,psi) -> Mux/4
  Demux/5 -> Extract x,y,psi4/1(s,n,psi,us)
  Extract x,y,psi4/1(x,y,psi) -> Mux/5
  s,n,psi,us (Cars 1 - 6)/1 -> Demux/1
  Mux/1 -> x,y,psi (Cars 1 - 6)/1
  Extract x,y,psi5/1(x,y,psi) -> Mux/6
  Demux/6 -> Extract x,y,psi5/1(s,n,psi,us)

== system template_Final_Project_MPC5643L/High-Level Design/Outputs/Subsystem ==
  Torque : Inport
  Add : Sum
  Constant : Constant  Value=0.5  OutDataTypeStr=single
  Constant1 : Constant  Value=0.0003162  OutDataTypeStr=single
  Constant2 : Constant  Value=20000  OutDataTypeStr=uint32
  Constant3 : Constant  Value=100  OutDataTypeStr=single
  Constant4 : Constant  Value=0  OutDataTypeStr=uint32
  Product : Product  RndMeth=Zero
  Product1 : Product  OutDataTypeStr=uint32  RndMeth=Zero
  Saturation : Saturate  UpperLimit=0.76  LowerLimit=0.24
  Simple PWM Output : rappid_564xl_ec_toolbox/MPC564xL/Motor Control Blocks/Simple PWM Output  Priority=1  pwmModule=0  pwmMod=0  SubModule=0  subMod=0  InitFreq=20000  resolution=1 %  resValue=1  InitDutyA=0  InitDutyB=0  align=A - edge aligned B - phase shifted  PhaseShift_A=0  PhaseShift=0  Phase_A=0  Phase_B=0  centered=-1  DoubleS=off  doubleSw=off  debugSw=off  debug_mode=0  pin_A0=None  pin_B0="59  : PD11 : [ 78 ] : [ R16 ]"  pin_X0=None  pin_A1=None  pin_B1=None  pin_X1=None  pin_A2=None  pin_B2=None  pin_X2=None  pin_A3=None  pin_B3=None  pin_X3=None  pin1_A0=None  pin1_B0=None  pin1_X0=None  pin1_A1=None  pin1_B1=None  pin1_X1=None  pin1_A2=None  pin1_B2=None  pin1_X2=None  pin1_A3=None  pin1_B3=None  pin1_X3=None  pcrNumA=255  pcrNumB=59  pcrNumX=255  polA=off  polB=off  polX=off  octrl=0  syncFrom0=off  masterSync=0  outVal0=off  outVal1=off  outVal2=on  outVal3=on  outVal4=on  outVal5=on  outTrig=60
  wires:
  Constant1/1 -> Product/2
  Torque/1 -> Product/1
  Product/1 -> Add/1
  Constant/1 -> Add/2
  Add/1 -> Saturation/1
  Constant2/1 -> Simple PWM Output/1
  Constant4/1 -> Simple PWM Output/4
  Saturation/1 -> Product1/1
  Product1/1 -> Simple PWM Output/2, Simple PWM Output/3
  Constant3/1 -> Product1/2

== system template_Final_Project_MPC5643L/High-Level Design/Outputs/Tx CAN ==
  s,n,psi,us : Inport
  CAN Transmit : rappid_564xl_ec_toolbox/MPC564xL/Communication Blocks/CAN Transmit  can_unit=A  can_unit_v2=0  can_buffer=0  can_id=45
  CAN Transmit1 : rappid_564xl_ec_toolbox/MPC564xL/Communication Blocks/CAN Transmit  can_unit=A  can_unit_v2=0  can_buffer=1  can_id=46
  Constant : Constant  Value=8  OutDataTypeStr=uint8
  Constant1 : Constant  Value=8  OutDataTypeStr=uint8
  Demux : Demux
  Mux : Mux  Inputs=2
  Mux1 : Mux  Inputs=2
  Single to Bytes{,1..3} (4 alike) : Conv_Lib/Single to Bytes
  wires:
  Constant1/1 -> CAN Transmit1/2
  Single to Bytes/1 -> Mux/1
  Single to Bytes1/1 -> Mux/2
  Single to Bytes2/1 -> Mux1/1
  Single to Bytes3/1 -> Mux1/2
  Mux/1 -> CAN Transmit/1
  Demux/1 -> Single to Bytes/1
  Demux/2 -> Single to Bytes1/1
  Demux/3 -> Single to Bytes3/1
  Demux/4 -> Single to Bytes2/1
  s,n,psi,us/1 -> Demux/1
  Constant/1 -> CAN Transmit/2
  Mux1/1 -> CAN Transmit1/1

== system template_Final_Project_MPC5643L/High-Level Design/Vehicle Model/Vehicle Dynamics ==
  Fd : Inport
  delta : Inport  Port=2
  Discrete-Time Integrator1 : DiscreteIntegrator  gainval=1  SampleTime=-1  ICPrevOutput=DiscIntNeverNeededParam  ICPrevScaledInput=DiscIntNeverNeededParam
  Discrete-Time Integrator2 : DiscreteIntegrator  gainval=1  SampleTime=-1  ICPrevOutput=DiscIntNeverNeededParam  ICPrevScaledInput=DiscIntNeverNeededParam
  Discrete-Time Integrator3 : DiscreteIntegrator  gainval=1  SampleTime=-1  ICPrevOutput=DiscIntNeverNeededParam  ICPrevScaledInput=DiscIntNeverNeededParam
  Discrete-Time Integrator4 : DiscreteIntegrator  gainval=1  SampleTime=-1  OutDataTypeStr=single  ICPrevOutput=DiscIntNeverNeededParam  ICPrevScaledInput=DiscIntNeverNeededParam
  Gain1 : Gain  Gain=1/m
  Gain4 : Gain  Gain=b
  S-Function Builder : S-Function  InitFcn=try, set_param(gcb,'FunctionName','vehicle_model'), end  FunctionName=vehicle_model  SFunctionModules=vehicle_model_wrapper  WizardData=DataTag1  EnableBusSupport=off  mask(S-Function Builder){}
      mask help: Simulink:masks:SFunctionBuilder_MD
      mask init: same as template_Final_Project_MPC5643L/High-Level Design/Vehicle Model/S-Function Builder
      settings: CopyFcn=set_param(gcbh,'LinkStatus','none')  PreSaveFcn=try, set_param(gcb,'FunctionName','vehicle_model'), end  OpenFcn=sfunctionwizard(gcbh)
      mask Display: plot(val(:,1),val(:,2)),disp(sys), port_label('input',1,'u'), port_label('input',2,'psi'), port_label('input',3,'delta'), port_label('output',1,'dotx'), port_label('output',2,'doty'), port_label('output',3,'dotpsi')
  Sum : Sum  Inputs=|+-
  x : Outport
  y : Outport  Port=2
  u : Outport  Port=3
  psi : Outport  Port=4
  wires:
  S-Function Builder/1 -> Discrete-Time Integrator1/1
  S-Function Builder/2 -> Discrete-Time Integrator2/1
  Sum/1 -> Gain1/1
  Gain1/1 -> Discrete-Time Integrator3/1
  Gain4/1 -> Sum/2
  Fd/1 -> Sum/1
  Discrete-Time Integrator3/1 -> u/1, S-Function Builder/1, Gain4/1
  Discrete-Time Integrator1/1 -> x/1
  Discrete-Time Integrator2/1 -> y/1
  S-Function Builder/3 -> Discrete-Time Integrator4/1
  Discrete-Time Integrator4/1 -> S-Function Builder/2, psi/1
  delta/1 -> S-Function Builder/3

== system template_Final_Project_MPC5643L/High-Level Design/Automatic Cruise Control/ACC_Subsystem/Subsystem ==
  s,n,psi,us (This Car) : Inport
  s,n,psi,us (Cars 1-6) : Inport  Port=2
  Fcn : Fcn  Expr=u(1)
  Fcn1 : Fcn  Expr=u(1)
  Fcn2 : Fcn  Expr=u(5)
  Fcn3 : Fcn  Expr=u(9)
  Fcn4 : Fcn  Expr=u(13)
  Fcn5 : Fcn  Expr=u(17)
  Fcn6 : Fcn  Expr=u(21)
  Mux1 : Mux  Inputs=7
  s : Outport
  wires:
  Fcn/1 -> Mux1/1
  Fcn4/1 -> Mux1/5
  Fcn3/1 -> Mux1/4
  Mux1/1 -> s/1
  Fcn5/1 -> Mux1/6
  Fcn2/1 -> Mux1/3
  Fcn1/1 -> Mux1/2
  s,n,psi,us (Cars 1-6)/1 -> Fcn3/1, Fcn4/1, Fcn5/1, Fcn6/1, Fcn2/1, Fcn1/1
  s,n,psi,us (This Car)/1 -> Fcn/1
  Fcn6/1 -> Mux1/7

== system template_Final_Project_MPC5643L/High-Level Design/Automatic Cruise Control/ACC_Subsystem/Subsystem1 ==
  s,n,psi,us (This Car) : Inport
  s,n,psi,us (Cars 1-6) : Inport  Port=2
  Fcn : Fcn  Expr=u(4)
  Fcn1 : Fcn  Expr=u(4)
  Fcn2 : Fcn  Expr=u(8)
  Fcn3 : Fcn  Expr=u(12)
  Fcn4 : Fcn  Expr=u(16)
  Fcn5 : Fcn  Expr=u(20)
  Fcn6 : Fcn  Expr=u(20)
  Mux1 : Mux  Inputs=7
  u : Outport
  wires:
  Fcn/1 -> Mux1/1
  Fcn4/1 -> Mux1/5
  Fcn3/1 -> Mux1/4
  Mux1/1 -> u/1
  Fcn5/1 -> Mux1/6
  Fcn2/1 -> Mux1/3
  Fcn1/1 -> Mux1/2
  s,n,psi,us (Cars 1-6)/1 -> Fcn3/1, Fcn4/1, Fcn5/1, Fcn6/1, Fcn2/1, Fcn1/1
  s,n,psi,us (This Car)/1 -> Fcn/1
  Fcn6/1 -> Mux1/7

== system template_Final_Project_MPC5643L/High-Level Design/Automatic Cruise Control/Speed Ctrl/PI ==
  Error : Inport
  Gain : Gain  Gain=V_Ki  SaturateOnIntegerOverflow=on  OutDataTypeStr=Inherit: Same as input  ParamDataTypeStr=Inherit: Same as input
  Gain1 : Gain  Gain=V_Kp  SaturateOnIntegerOverflow=on  OutDataTypeStr=Inherit: Same as input  ParamDataTypeStr=Inherit: Same as input
  My Discrete Integrator : Subsystem
  Sum : Sum  Inputs=|++  SaturateOnIntegerOverflow=on
  U : Outport
  wires:
  Sum/1 -> U/1
  Error/1 -> Gain1/1, Gain/1
  Gain1/1 -> Sum/2
  My Discrete Integrator/1(X) -> Sum/1
  Gain/1 -> My Discrete Integrator/1(X_dot)

== system template_Final_Project_MPC5643L/High-Level Design/Automatic Steering/Automatic Steering/derivative ==
  In : Inport
  Gain5 : Gain  Gain=1/dT
  Sum4 : Sum  Inputs=|+-
  Unit Delay : UnitDelay  SampleTime=-1
  Out : Outport
  wires:
  Sum4/1 -> Gain5/1
  Unit Delay/1 -> Sum4/2
  In/1 -> Sum4/1, Unit Delay/1
  Gain5/1 -> Out/1

== system template_Final_Project_MPC5643L/High-Level Design/Automatic Steering/Automatic Steering/derivative1 ==
  In : Inport
  Gain5 : Gain  Gain=1/dT
  Sum4 : Sum  Inputs=|+-
  Unit Delay : UnitDelay  SampleTime=-1
  Out : Outport
  wires:
  Sum4/1 -> Gain5/1
  Unit Delay/1 -> Sum4/2
  In/1 -> Sum4/1, Unit Delay/1
  Gain5/1 -> Out/1

== system template_Final_Project_MPC5643L/High-Level Design/Inputs/Haptic Wheel Input/Subsystem ==
  encoder counts : Inport
  Data Type Conversion : DataTypeConversion  OutDataTypeStr=uint16
  Data Type Conversion1 : DataTypeConversion  OutDataTypeStr=int16
  Data Type Conversion2 : DataTypeConversion  OutDataTypeStr=single
  Gain : Gain  Gain=0.00157080
  Sum : Sum  Inputs=|+-
  Sum1 : Sum  Inputs=|++
  Unit Delay : UnitDelay  SampleTime=-1
  Unit Delay1 : UnitDelay  SampleTime=-1
  Haptic  Wheel  Position  (radians) : Outport
  wires:
  encoder counts/1 -> Data Type Conversion/1
  Data Type Conversion/1 -> Sum/1, Unit Delay/1
  Sum/1 -> Data Type Conversion1/1
  Unit Delay/1 -> Sum/2
  Data Type Conversion1/1 -> Data Type Conversion2/1
  Data Type Conversion2/1 -> Gain/1
  Gain/1 -> Sum1/1
  Unit Delay1/1 -> Sum1/2
  Sum1/1 -> Haptic  Wheel  Position  (radians)/1, Unit Delay1/1

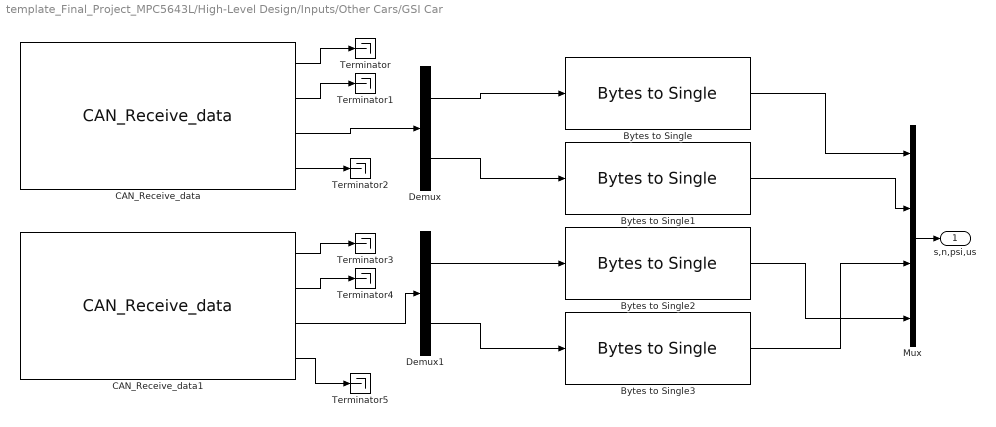
== system template_Final_Project_MPC5643L/High-Level Design/Inputs/Other Cars/GSI Car ==
  Bytes to Single{,1..3} (4 alike) : Conv_Lib/Bytes to Single
  CAN_Receive_data : rappid_564xl_ec_toolbox/MPC564xL/Communication Blocks/CAN_Receive_data  can_unit=A  can_unit_v2=0  can_buffer=12  can_id=15
  CAN_Receive_data1 : rappid_564xl_ec_toolbox/MPC564xL/Communication Blocks/CAN_Receive_data  can_unit=A  can_unit_v2=0  can_buffer=13  can_id=16
  Demux : Demux  Outputs=2
  Demux1 : Demux  Outputs=2
  Mux : Mux
  Terminator{,1..5} (6 alike) : Terminator
  s,n,psi,us : Outport
  wires:
  Bytes to Single1/1 -> Mux/2
  Bytes to Single3/1 -> Mux/3
  Demux/1 -> Bytes to Single/1
  Demux/2 -> Bytes to Single1/1
  Demux1/1 -> Bytes to Single2/1
  Demux1/2 -> Bytes to Single3/1
  Bytes to Single/1 -> Mux/1
  Bytes to Single2/1 -> Mux/4
  Mux/1 -> s,n,psi,us/1
  CAN_Receive_data/1 -> Terminator/1
  CAN_Receive_data/2 -> Terminator1/1
  CAN_Receive_data/3 -> Demux/1
  CAN_Receive_data/4 -> Terminator2/1
  CAN_Receive_data1/1 -> Terminator3/1
  CAN_Receive_data1/2 -> Terminator4/1
  CAN_Receive_data1/3 -> Demux1/1
  CAN_Receive_data1/4 -> Terminator5/1

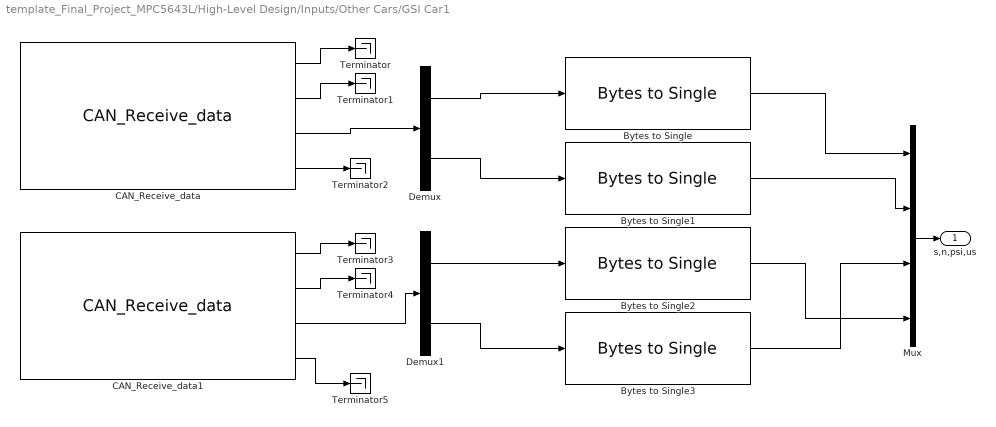
== system template_Final_Project_MPC5643L/High-Level Design/Inputs/Other Cars/GSI Car1 ==
  Bytes to Single{,1..3} (4 alike) : Conv_Lib/Bytes to Single
  CAN_Receive_data : rappid_564xl_ec_toolbox/MPC564xL/Communication Blocks/CAN_Receive_data  can_unit=A  can_unit_v2=0  can_buffer=2  can_id=35
  CAN_Receive_data1 : rappid_564xl_ec_toolbox/MPC564xL/Communication Blocks/CAN_Receive_data  can_unit=A  can_unit_v2=0  can_buffer=3  can_id=36
  Demux : Demux  Outputs=2
  Demux1 : Demux  Outputs=2
  Mux : Mux
  Terminator{,1..5} (6 alike) : Terminator
  s,n,psi,us : Outport
  wires:
  Bytes to Single1/1 -> Mux/2
  Bytes to Single3/1 -> Mux/3
  Demux/1 -> Bytes to Single/1
  Demux/2 -> Bytes to Single1/1
  Demux1/1 -> Bytes to Single2/1
  Demux1/2 -> Bytes to Single3/1
  Bytes to Single/1 -> Mux/1
  Bytes to Single2/1 -> Mux/4
  Mux/1 -> s,n,psi,us/1
  CAN_Receive_data/1 -> Terminator/1
  CAN_Receive_data/2 -> Terminator1/1
  CAN_Receive_data/3 -> Demux/1
  CAN_Receive_data/4 -> Terminator2/1
  CAN_Receive_data1/1 -> Terminator3/1
  CAN_Receive_data1/2 -> Terminator4/1
  CAN_Receive_data1/3 -> Demux1/1
  CAN_Receive_data1/4 -> Terminator5/1

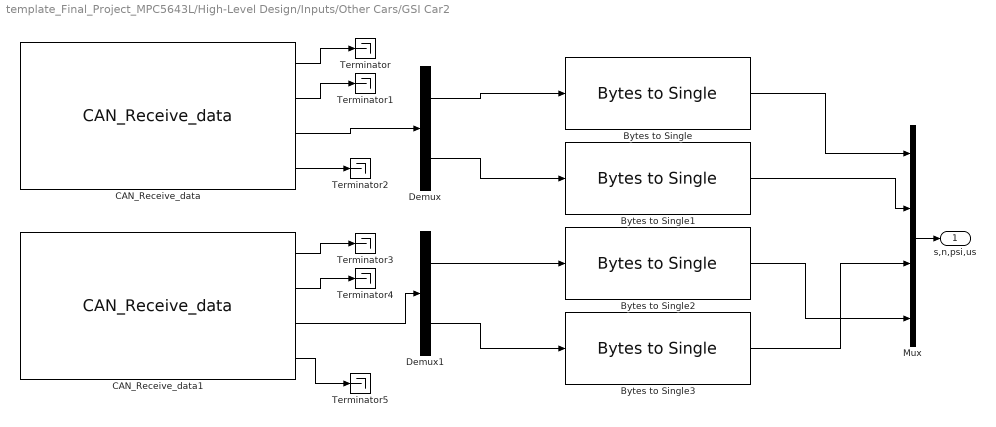
== system template_Final_Project_MPC5643L/High-Level Design/Inputs/Other Cars/GSI Car2 ==
  Bytes to Single{,1..3} (4 alike) : Conv_Lib/Bytes to Single
  CAN_Receive_data : rappid_564xl_ec_toolbox/MPC564xL/Communication Blocks/CAN_Receive_data  can_unit=A  can_unit_v2=0  can_buffer=4  can_id=25
  CAN_Receive_data1 : rappid_564xl_ec_toolbox/MPC564xL/Communication Blocks/CAN_Receive_data  can_unit=A  can_unit_v2=0  can_buffer=5  can_id=26
  Demux : Demux  Outputs=2
  Demux1 : Demux  Outputs=2
  Mux : Mux
  Terminator{,1..5} (6 alike) : Terminator
  s,n,psi,us : Outport
  wires:
  Bytes to Single1/1 -> Mux/2
  Bytes to Single3/1 -> Mux/3
  Demux/1 -> Bytes to Single/1
  Demux/2 -> Bytes to Single1/1
  Demux1/1 -> Bytes to Single2/1
  Demux1/2 -> Bytes to Single3/1
  Bytes to Single/1 -> Mux/1
  Bytes to Single2/1 -> Mux/4
  Mux/1 -> s,n,psi,us/1
  CAN_Receive_data/1 -> Terminator/1
  CAN_Receive_data/2 -> Terminator1/1
  CAN_Receive_data/3 -> Demux/1
  CAN_Receive_data/4 -> Terminator2/1
  CAN_Receive_data1/1 -> Terminator3/1
  CAN_Receive_data1/2 -> Terminator4/1
  CAN_Receive_data1/3 -> Demux1/1
  CAN_Receive_data1/4 -> Terminator5/1

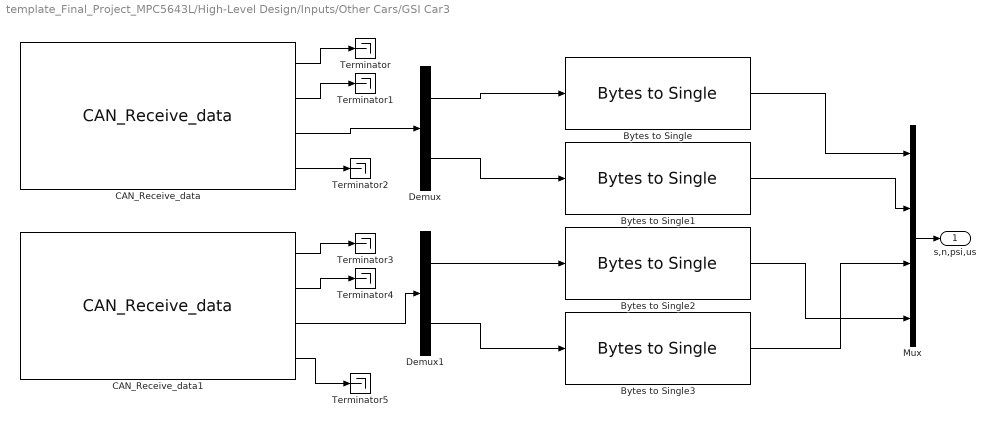
== system template_Final_Project_MPC5643L/High-Level Design/Inputs/Other Cars/GSI Car3 ==
  Bytes to Single{,1..3} (4 alike) : Conv_Lib/Bytes to Single
  CAN_Receive_data : rappid_564xl_ec_toolbox/MPC564xL/Communication Blocks/CAN_Receive_data  can_unit=A  can_unit_v2=0  can_buffer=6  can_id=55
  CAN_Receive_data1 : rappid_564xl_ec_toolbox/MPC564xL/Communication Blocks/CAN_Receive_data  can_unit=A  can_unit_v2=0  can_buffer=7  can_id=56
  Demux : Demux  Outputs=2
  Demux1 : Demux  Outputs=2
  Mux : Mux
  Terminator{,1..5} (6 alike) : Terminator
  s,n,psi,us : Outport
  wires:
  Bytes to Single1/1 -> Mux/2
  Bytes to Single3/1 -> Mux/3
  Demux/1 -> Bytes to Single/1
  Demux/2 -> Bytes to Single1/1
  Demux1/1 -> Bytes to Single2/1
  Demux1/2 -> Bytes to Single3/1
  Bytes to Single/1 -> Mux/1
  Bytes to Single2/1 -> Mux/4
  Mux/1 -> s,n,psi,us/1
  CAN_Receive_data/1 -> Terminator/1
  CAN_Receive_data/2 -> Terminator1/1
  CAN_Receive_data/3 -> Demux/1
  CAN_Receive_data/4 -> Terminator2/1
  CAN_Receive_data1/1 -> Terminator3/1
  CAN_Receive_data1/2 -> Terminator4/1
  CAN_Receive_data1/3 -> Demux1/1
  CAN_Receive_data1/4 -> Terminator5/1

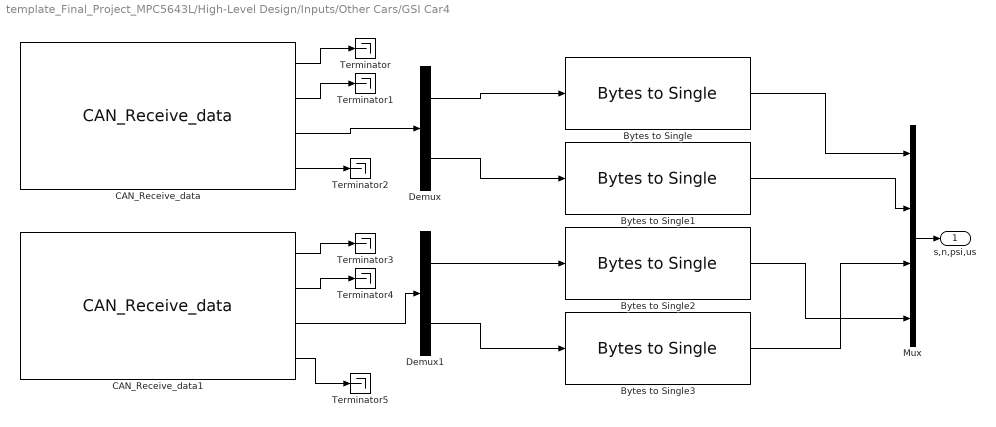
== system template_Final_Project_MPC5643L/High-Level Design/Inputs/Other Cars/GSI Car4 ==
  Bytes to Single{,1..3} (4 alike) : Conv_Lib/Bytes to Single
  CAN_Receive_data : rappid_564xl_ec_toolbox/MPC564xL/Communication Blocks/CAN_Receive_data  can_unit=A  can_unit_v2=0  can_buffer=8  can_id=65
  CAN_Receive_data1 : rappid_564xl_ec_toolbox/MPC564xL/Communication Blocks/CAN_Receive_data  can_unit=A  can_unit_v2=0  can_buffer=9  can_id=66
  Demux : Demux  Outputs=2
  Demux1 : Demux  Outputs=2
  Mux : Mux
  Terminator{,1..5} (6 alike) : Terminator
  s,n,psi,us : Outport
  wires:
  Bytes to Single1/1 -> Mux/2
  Bytes to Single3/1 -> Mux/3
  Demux/1 -> Bytes to Single/1
  Demux/2 -> Bytes to Single1/1
  Demux1/1 -> Bytes to Single2/1
  Demux1/2 -> Bytes to Single3/1
  Bytes to Single/1 -> Mux/1
  Bytes to Single2/1 -> Mux/4
  Mux/1 -> s,n,psi,us/1
  CAN_Receive_data/1 -> Terminator/1
  CAN_Receive_data/2 -> Terminator1/1
  CAN_Receive_data/3 -> Demux/1
  CAN_Receive_data/4 -> Terminator2/1
  CAN_Receive_data1/1 -> Terminator3/1
  CAN_Receive_data1/2 -> Terminator4/1
  CAN_Receive_data1/3 -> Demux1/1
  CAN_Receive_data1/4 -> Terminator5/1

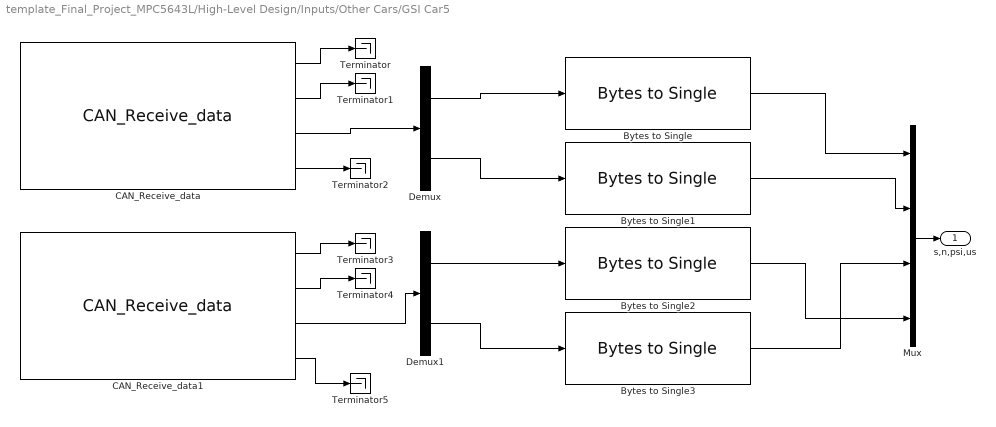
== system template_Final_Project_MPC5643L/High-Level Design/Inputs/Other Cars/GSI Car5 ==
  Bytes to Single{,1..3} (4 alike) : Conv_Lib/Bytes to Single
  CAN_Receive_data : rappid_564xl_ec_toolbox/MPC564xL/Communication Blocks/CAN_Receive_data  can_unit=A  can_unit_v2=0  can_buffer=10  can_id=75
  CAN_Receive_data1 : rappid_564xl_ec_toolbox/MPC564xL/Communication Blocks/CAN_Receive_data  can_unit=A  can_unit_v2=0  can_buffer=11  can_id=76
  Demux : Demux  Outputs=2
  Demux1 : Demux  Outputs=2
  Mux : Mux
  Terminator{,1..5} (6 alike) : Terminator
  s,n,psi,us : Outport
  wires:
  Bytes to Single1/1 -> Mux/2
  Bytes to Single3/1 -> Mux/3
  Demux/1 -> Bytes to Single/1
  Demux/2 -> Bytes to Single1/1
  Demux1/1 -> Bytes to Single2/1
  Demux1/2 -> Bytes to Single3/1
  Bytes to Single/1 -> Mux/1
  Bytes to Single2/1 -> Mux/4
  Mux/1 -> s,n,psi,us/1
  CAN_Receive_data/1 -> Terminator/1
  CAN_Receive_data/2 -> Terminator1/1
  CAN_Receive_data/3 -> Demux/1
  CAN_Receive_data/4 -> Terminator2/1
  CAN_Receive_data1/1 -> Terminator3/1
  CAN_Receive_data1/2 -> Terminator4/1
  CAN_Receive_data1/3 -> Demux1/1
  CAN_Receive_data1/4 -> Terminator5/1

== system template_Final_Project_MPC5643L/High-Level Design/Outputs/Extract x,y,psi (Cars 1 - 6)/Extract x,y,psi ==
  s,n,psi,us : Inport
  Demux : Demux
  Mux : Mux  Inputs=3
  Terminator : Terminator
  s,n to x,y : Veh_Sim/s,n to x,y  SystemSampleTime=-1
  x,y,psi : Outport
  wires:
  Demux/1 -> s,n to x,y/1
  Demux/2 -> s,n to x,y/2
  s,n,psi,us/1 -> Demux/1
  s,n to x,y/1 -> Mux/1
  s,n to x,y/2 -> Mux/2
  Demux/3 -> Mux/3
  Mux/1 -> x,y,psi/1
  Demux/4 -> Terminator/1

== system template_Final_Project_MPC5643L/High-Level Design/Outputs/Extract x,y,psi (Cars 1 - 6)/Extract x,y,psi1 ==
  s,n,psi,us : Inport
  Demux : Demux
  Mux : Mux  Inputs=3
  Terminator : Terminator
  s,n to x,y : Veh_Sim/s,n to x,y  SystemSampleTime=-1
  x,y,psi : Outport
  wires:
  Demux/1 -> s,n to x,y/1
  Demux/2 -> s,n to x,y/2
  s,n,psi,us/1 -> Demux/1
  s,n to x,y/1 -> Mux/1
  s,n to x,y/2 -> Mux/2
  Demux/3 -> Mux/3
  Mux/1 -> x,y,psi/1
  Demux/4 -> Terminator/1

== system template_Final_Project_MPC5643L/High-Level Design/Outputs/Extract x,y,psi (Cars 1 - 6)/Extract x,y,psi2 ==
  s,n,psi,us : Inport
  Demux : Demux
  Mux : Mux  Inputs=3
  Terminator : Terminator
  s,n to x,y : Veh_Sim/s,n to x,y  SystemSampleTime=-1
  x,y,psi : Outport
  wires:
  Demux/1 -> s,n to x,y/1
  Demux/2 -> s,n to x,y/2
  s,n,psi,us/1 -> Demux/1
  s,n to x,y/1 -> Mux/1
  s,n to x,y/2 -> Mux/2
  Demux/3 -> Mux/3
  Mux/1 -> x,y,psi/1
  Demux/4 -> Terminator/1

== system template_Final_Project_MPC5643L/High-Level Design/Outputs/Extract x,y,psi (Cars 1 - 6)/Extract x,y,psi3 ==
  s,n,psi,us : Inport
  Demux : Demux
  Mux : Mux  Inputs=3
  Terminator : Terminator
  s,n to x,y : Veh_Sim/s,n to x,y  SystemSampleTime=-1
  x,y,psi : Outport
  wires:
  Demux/1 -> s,n to x,y/1
  Demux/2 -> s,n to x,y/2
  s,n,psi,us/1 -> Demux/1
  s,n to x,y/1 -> Mux/1
  s,n to x,y/2 -> Mux/2
  Demux/3 -> Mux/3
  Mux/1 -> x,y,psi/1
  Demux/4 -> Terminator/1

== system template_Final_Project_MPC5643L/High-Level Design/Outputs/Extract x,y,psi (Cars 1 - 6)/Extract x,y,psi4 ==
  s,n,psi,us : Inport
  Demux : Demux
  Mux : Mux  Inputs=3
  Terminator : Terminator
  s,n to x,y : Veh_Sim/s,n to x,y  SystemSampleTime=-1
  x,y,psi : Outport
  wires:
  Demux/1 -> s,n to x,y/1
  Demux/2 -> s,n to x,y/2
  s,n,psi,us/1 -> Demux/1
  s,n to x,y/1 -> Mux/1
  s,n to x,y/2 -> Mux/2
  Demux/3 -> Mux/3
  Mux/1 -> x,y,psi/1
  Demux/4 -> Terminator/1
